simulink model "cart_2"  (R2022a)
settings: Solver=FixedStepAuto  StartTime=0.0  StopTime=10.0  FixedStep=0.01  RelTol=1e-3
settings Model: Creator=Home  LastModifiedBy=Home

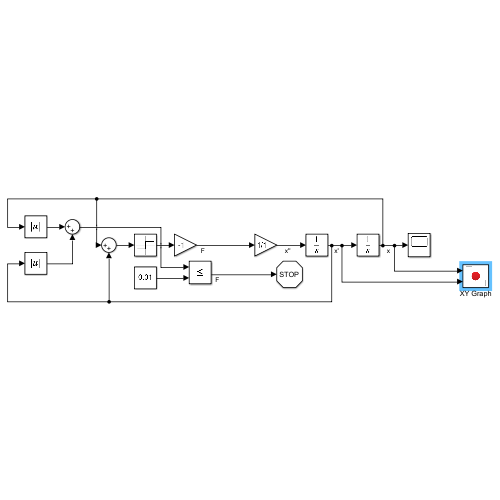
[thumbnail: Simulink's stored preview of the top-level diagram]
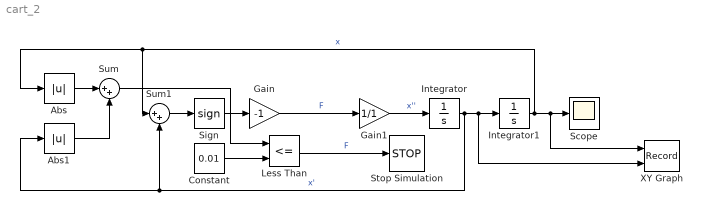
== system cart_2 ==
  Abs : Abs  SaturateOnIntegerOverflow=off
  Abs1 : Abs  SaturateOnIntegerOverflow=off
  Constant : Constant  Value=0.01
  Gain : Gain  Gain=-1
  Gain1 : Gain  Gain=1/1
  Integrator : Integrator
  Integrator1 : Integrator  InitialCondition=1
  Less Than : RelationalOperator  Operator=<=  OutDataTypeStr=boolean  RndMeth=Simplest  InputSameDT=off
  Scope : Scope
  Sign : Signum
  Stop Simulation : Stop
  Sum : Sum  Inputs=|++
  Sum1 : Sum  Inputs=|++
  XY Graph : Record  FileSettingsInternal="{\"entries\":[{\"content\":{\"excelSettings\":{\"content\":{},\"type\":\"Streamout.ExcelSettings\"}},\"type\":\"Streamout.FileSettingStorage\",\"uuid\":\"6f19eb96-6070-4a0a-bb22-1de6dda950e3\"}],\"packageUris\":[\"http://schema.mathworks.com/mf0/streamout_blocks/R2020a\"],\"version\":\"1.0\"}"  Layout=[1 1]  SignalsInternal="{\"entries\":[{\"content\":{\"signals\":[{\"content\":{\"blockPath\":[\"cart_2/XY Graph\"],\"channel\":[],\"dimensions\":[1],\"domain\":\"cart_2/XY Graph\",\"lineColor\":\"#a2142f\",\"plots\":[1],\"port\":1,\"sid\":[\"\"],\"signalID\":117,\"signalName\":\"x\"},\"type\":\"RecordBlkView.Signal\",\"uuid\":\"202c426b-5694-4288-87bd-3e18c6d869fd\"},{\"content\":{\"blockPath\":[\"cart_2/XY Graph\"],\"channel\":[],\"dimensions\":[1],\"domain\":\"cart_2/XY Graph\",\"lineColor\":\"#139fff\",\"plots\":[1],\"port\":2,\"sid\":[\"\"],\"signalID\":121,\"signalName\":\"x'\"},\"type\":\"RecordBlkView.Signal\",\"uuid\":\"39f9f44c-f225-4c23-9fa3-cc3fce6f8ead\"}]},\"type\":\"RecordBlkView.InputSignals\",\"uuid\":\"52e427ea-0084-40d1-a456-de2010d4607f\"}],\"packageUris\":[\"http://schema.mathworks.com/mf0/streamout_blocks/R2020a\"],\"version\":\"1.0\"}"  VisualizationBindings="{\"xyplotplugin\":{\"info\":[{\"series\":[{\"bindingParametersList\":[{\"parameter\":\"X-Axis\",\"signalID\":117,\"signalName\":\"x\"},{\"parameter\":\"Y-Axis\",\"signalID\":121,\"signalName\":\"x'\"}],\"seriesID\":42633}],\"subplotID\":1}]}}"  CompatibilityTag=XY
  wires:
  Integrator/1 -> Abs1/1, Sum1/2, XY Graph/2, Integrator1/1  "x'"
  Integrator1/1 -> Sum1/1, Abs/1, XY Graph/1, Scope/1  "x"
  Gain1/1 -> Integrator/1  "x''"
  Abs/1 -> Sum/1
  Abs1/1 -> Sum/2
  Sum/1 -> Less Than/1
  Constant/1 -> Less Than/2
  Sum1/1 -> Sign/1
  Sign/1 -> Gain/1
  Gain/1 -> Gain1/1  "F"
  Less Than/1 -> Stop Simulation/1  "F"
